simulink model "verify_Flow_Mixer_basic_mdl"  (R2018b)
settings: Solver=VariableStepDiscrete  StartTime=0.0  StopTime=10.0  MaxStep=0.1  RelTol=1e-3  EnableMultiTasking=on
libraries: carnot x5
settings Model: Creator=drhf  LastModifiedBy=drhf
settings DataIOCC: LimitDataPoints=on  SaveFormat=Array
settings OptimizationCC: ExpressionDepthLimit=2147483647  LifeSpan=inf
settings DebuggingCC: UnderspecifiedInitializationDetection=Classic  MergeDetectMultiDrivingBlocksExec=none  SolverPrmCheckMsg=warning  StateNameClashWarn=warning  SFUnexpectedBacktrackingDiag=warning  SFNoUnconditionalDefaultTransitionDiag=warning  SFExecutionAtInitializationDiag=none
settings HardwareCC: ProdBitPerPointer=32  ProdBitPerSizeT=32  ProdBitPerPtrDiffT=32  ProdLargestAtomicFloat=None  ProdIntDivRoundTo=Undefined  ProdEndianess=Unspecified  ProdWordSize=32  ProdHWDeviceType=32-bit Generic
settings ModelReferenceCC: PropagateSignalLabelsOutOfModel=off
settings SFSimCC: SimUseLocalCustomCode=off
settings RTWCC: RTWUseLocalCustomCode=off
settings CodeAppCC: StateflowObjectComments=on
settings GRTTargetCC: TargetLangStandard=C89/C90 (ANSI)  GeneratePreprocessorConditionals=Disable all  CombineOutputUpdateFcns=off  GRTInterface=on
settings ConfigComp: CovMetricSettings=dw  CovHtmlReporting=on  CovSaveCumulativeToWorkspaceVar=on  CovSaveSingleToWorkspaceVar=on  CovExternalEMLEnable=off

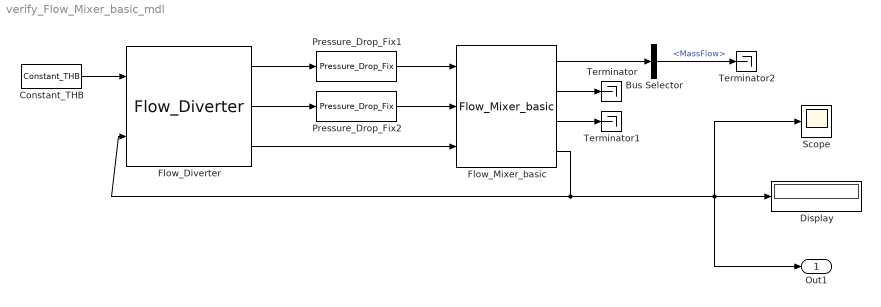
== system verify_Flow_Mixer_basic_mdl ==
  Bus Selector : BusSelector  OutputSignals=MassFlow
  Constant_THB : carnot/Source/Simple/Constant_THB  t=40  mdot=1  p=1e5  mID=No Pressure Drop  fluid=Water  mix=0  mix2=0  mix3=0  dia=0.1  hgt=0
  Display : Display
  Flow_Diverter : carnot/Hydraulics/Flow_Diverter
  Flow_Mixer_basic : carnot/Basic/Hydraulics/Flow_Mixer_basic
  Pressure_Drop_Fix1 : carnot/Basic/Pressure_Drop/Pressure_Drop_Fix  con=0  lin=10  qua=0
  Pressure_Drop_Fix2 : carnot/Basic/Pressure_Drop/Pressure_Drop_Fix  con=0  lin=20  qua=0
  Scope : Scope
  Terminator : Terminator
  Terminator1 : Terminator
  Terminator2 : Terminator
  Out1 : Outport
  wires:
  Flow_Mixer_basic/4 -> Scope/1, Out1/1, Display/1, Flow_Diverter/2
  Flow_Diverter/1 -> Pressure_Drop_Fix1/1
  Flow_Diverter/2 -> Pressure_Drop_Fix2/1
  Constant_THB/1 -> Flow_Diverter/1
  Flow_Diverter/3 -> Flow_Mixer_basic/3
  Flow_Mixer_basic/2 -> Terminator/1
  Flow_Mixer_basic/3 -> Terminator1/1
  Pressure_Drop_Fix1/1 -> Flow_Mixer_basic/1
  Pressure_Drop_Fix2/1 -> Flow_Mixer_basic/2
  Flow_Mixer_basic/1 -> Bus Selector/1
  Bus Selector/1 -> Terminator2/1  "<MassFlow>"
